simulink model "temp_model"  (R2021a)
settings: Solver=VariableStepAuto  StartTime=0.0  StopTime=10.0  RelTol=1e-3
settings Model: Creator=DELL  LastModifiedBy=DELL

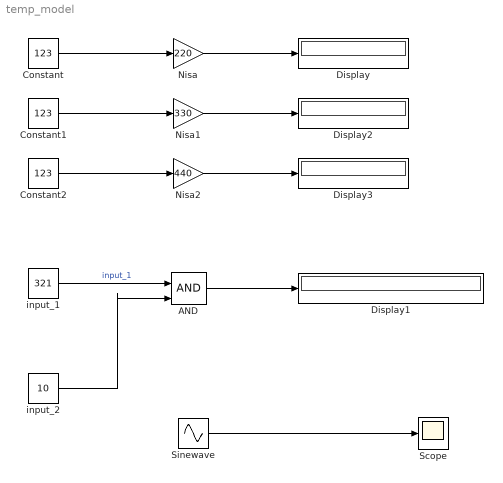
== system temp_model ==
  AND : Logic  IconShape=distinctive  AllPortsSameDT=off  OutDataTypeStr=boolean
  Constant : Constant  Value=123
  Constant1 : Constant  Value=123
  Constant2 : Constant  Value=123
  Display{,1..3} (4 alike) : Display
      Display1 settings: Decimation=12323
  Nisa : Gain  Gain=220
  Nisa1 : Gain  Gain=330
  Nisa2 : Gain  Gain=440
  Scope : Scope
  Sinewave : Sin  Amplitude=5  SampleTime=0
  input_1 : Constant  Value=321
  input_2 : Constant  Value=10
  wires:
  Constant/1 -> Nisa/1
  Nisa/1 -> Display/1
  AND/1 -> Display1/1
  input_2/1 -> AND/2
  input_1/1 -> AND/1  "input_1"
  Sinewave/1 -> Scope/1
  Nisa1/1 -> Display2/1
  Constant1/1 -> Nisa1/1
  Constant2/1 -> Nisa2/1
  Nisa2/1 -> Display3/1
